simulink model "accelerate"  (R2022a)
settings: Solver=VariableStepAuto  StartTime=0.0  StopTime=2  FixedStep=0.0001  RelTol=1e-2  AbsTol=1e-2  EnableMultiTasking=on
InitFcn:
  | run('parameters.m')
  | run('initBusObjects.m')
  | run('loadTrajectory.m')
settings Model: Creator=chrismailer  LastModifiedBy=chrismailer
settings SolverCC: AutoScaleAbsTol=off  NumberNewtonIterations=3  ZeroCrossAlgorithm=Adaptive  AlgebraicLoopSolver=TrustRegion  AutoInsertRateTranBlk=on
settings DataIOCC: LimitDataPoints=on  MaxDataPoints=10000
settings OptimizationCC: LifeSpan=inf
settings DebuggingCC: UnconnectedInputMsg=warning  UnconnectedOutputMsg=warning  UnconnectedLineMsg=warning  AllowSymbolicDim=off  SFUnexpectedBacktrackingDiag=warning  SFNoUnconditionalDefaultTransitionDiag=warning  SFExecutionAtInitializationDiag=none  SFMachineParentedDataDiag=warning  ArithmeticOperatorsInVariantConditions=warning
settings SFSimCC: SimUseLocalCustomCode=off  CustomCodeUndefinedFunction=UseInterfaceOnly
settings RTWCC: RTWUseLocalCustomCode=off  DLArmComputeVersion=19.05
settings CodeAppCC: StateflowObjectComments=on
settings GRTTargetCC: TargetLangStandard=C89/C90 (ANSI)
settings ConfigComp: CovMetricSettings=dw  CovSaveCumulativeToWorkspaceVar=on  CovSaveSingleToWorkspaceVar=on  CovExternalEMLEnable=off  CovSFcnEnable=off
settings SimscapeCC: SimscapeLogType=all  SimscapeLogSimulationStatistics=on  SimscapeLogDataHistory=10000
settings ExplorerConfigSet: InternalSimMechanicsExplorerSettings="<ExplorerConfiguration><canonicalview>default</canonicalview><AnimationSetting><BasePlaybackSpeed>1.0</BasePlaybackSpeed><PlaybackSpeedFactor>0.125</PlaybackSpeedFactor></AnimationSetting><TilePanel><TileInfo><Tiles Columns=\"1\" Count=\"1\" Rows=\"1\"><Column Weight=\"1\"/><Row Weight=\"1\"/><Tile Height=\"1\" Width=\"1\" X=\"0\" Y=\"0\"/></Tiles></TileInfo><SceneInfo><SceneViewer><BGColor><R>1</R><G>1</G><B>1</B></BGColor><Camera><DoPerspective>on</DoPerspective><Position><X>3.29782276099316451</X><Y>0.285165922205473821</Y><Z>0.279114537761918247</Z></Position><Center><X>2.60042520557901913</X><Y>0.224861281402514157</Y><Z>0.27911453776191808</Z></Center><Up><X>0</X><Y>0</Y><Z>1</Z></Up><ViewLimDist>1</ViewLimDist><YLim>0.466307658154998583</YLim><XLim>0.737672809220199066</XLim></Camera></SceneViewer></SceneInfo></TilePanel><MechEditorPanel><Cameras><Camera><Id>Camera1</Id><Value><Name>Camera1</Name><NativeCamera><PositionTrackingFeature>Kemba_Simulation.Camera_Origin.R</PositionTrackingFeature><CenterTrackingFeature>Kemba_Simulation.Body.R</CenterTrackingFeature><UpVectorTrackingFeature>Kemba_Simulation.World_Frame.W</UpVectorTrackingFeature><CenterTrackingOrigin>on</CenterTrackingOrigin><UpVectorTrackingDirection>+Z</UpVectorTrackingDirection></NativeCamera></Value></Camera></Cameras><GfxPanelCameraMap><MapElement CameraMLId=\"Camera1\" GfxPanelIndex=\"0\"/></GfxPanelCameraMap><VideoCreator><PlaybackSpeedRatio>1.0</PlaybackSpeedRatio><FrameRate>30</FrameRate><VideoFormat>MPEG-4</VideoFormat><FrameSize>[1920 1080]</FrameSize></VideoCreator></MechEditorPanel></ExplorerConfiguration>"

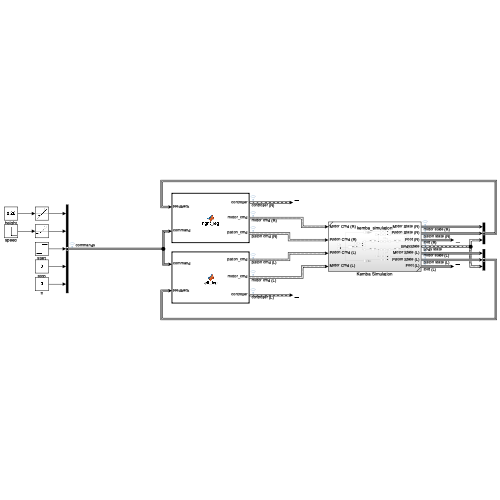
[thumbnail: Simulink's stored preview of the top-level diagram]
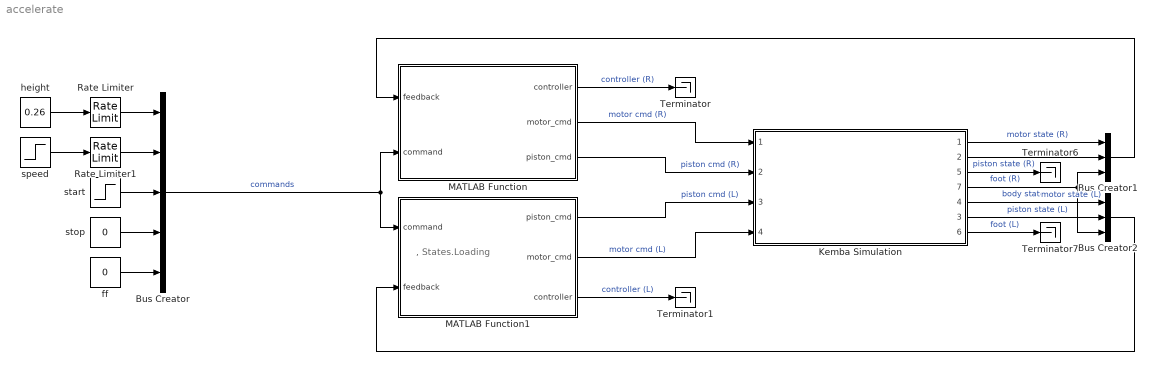
== system accelerate ==
  note: , States.Loading
  Bus Creator : BusCreator  Inputs=5  OutDataTypeStr=Bus: Command
      settings: InheritFromInputs=off
  Bus Creator1 : BusCreator  Inputs=3  OutDataTypeStr=Bus: State
      settings: InheritFromInputs=off
  Bus Creator2 : BusCreator  Inputs=3  OutDataTypeStr=Bus: State
      settings: InheritFromInputs=off
  Kemba Simulation : Subsystem  ReferencedSubsystem=kemba_simulation
      settings: PortSchema="{\"entries\":[{\"content\":{\"sides\":[{\"content\":{\"connectorIds\":[\"In1\",\"In2\",\"In3\",\"In4\"]},\"type\":\"ConnectorPlacement.EquallySpacedRectSide\",\"uuid\":\"35a785e7-99ad-4766-87e3-a239e5d8a8f8\"},{\"content\":{\"connectorIds\":[\"Out1\",\"Out2\",\"Out5\",\"Out7\",\"Out4\",\"Out3\",\"Out6\"],\"side\":\"RIGHT\"},\"type\":\"ConnectorPlacement.EquallySpacedRectSide\",\"uuid\":\"8c5f00f3-e1d5-4c02-a562-5da7bf8e4c30\"},{\"content\":{\"connectorIds\":[],\"side\":\"TOP\"},\"type\":\"ConnectorPlacement.EquallySpacedRectSide\",\"uuid\":\"cf7efd56-02a7-4dc2-b997-d6a0137d575f\"}]},\"type\":\"ConnectorPlacement.EquallySpacedConnector\",\"uuid\":\"7dd37b2d-e40a-4db8-86aa-8036efc7fb4f\"}],\"packageUris\":[\"http://schema.mathworks.com/mf0/Connector/R2020b\"],\"version\":\"1.0\"}"
  MATLAB Function : MATLAB Function  TreatAsAtomicUnit=on  SystemSampleTime=0.001
  MATLAB Function1 : MATLAB Function  TreatAsAtomicUnit=on  SystemSampleTime=0.001
  Rate Limiter : RateLimiter  RisingSlewLimit=0.05  FallingSlewLimit=-0.05  SampleTimeMode=inherited
  Rate Limiter1 : RateLimiter  RisingSlewLimit=0.4  FallingSlewLimit=-0.4  SampleTimeMode=inherited  InitialCondition=1.5
  Terminator{,1,6..7} (4 alike) : Terminator
  ff : Constant  Value=0
  height : Constant  Value=0.26
  speed : Step  Time=2  Before=1.5  After=0  SampleTime=0
  start : Step  Time=0.5  SampleTime=0
  stop : Constant  Value=0
  wires:
  MATLAB Function/2(motor_cmd) -> Kemba Simulation/1  "motor cmd (R)"
  Kemba Simulation/7 -> Bus Creator2/3, Bus Creator1/3  "body state"
  MATLAB Function/3(piston_cmd) -> Kemba Simulation/2  "piston cmd (R)"
  MATLAB Function1/2(motor_cmd) -> Kemba Simulation/4  "motor cmd (L)"
  MATLAB Function/1(controller) -> Terminator/1  "controller (R)"
  MATLAB Function1/3(controller) -> Terminator1/1  "controller (L)"
  height/1 -> Rate Limiter/1
  MATLAB Function1/1(piston_cmd) -> Kemba Simulation/3  "piston cmd (L)"
  Kemba Simulation/2 -> Bus Creator1/2  "piston state (R)"
  Kemba Simulation/1 -> Bus Creator1/1  "motor state (R)"
  Bus Creator1/1 -> MATLAB Function/1(feedback)
  Kemba Simulation/3 -> Bus Creator2/2  "piston state (L)"
  Kemba Simulation/4 -> Bus Creator2/1  "motor state (L)"
  Bus Creator2/1 -> MATLAB Function1/2(feedback)
  start/1 -> Bus Creator/3
  Kemba Simulation/5 -> Terminator6/1  "foot (R)"
  Kemba Simulation/6 -> Terminator7/1  "foot (L)"
  Rate Limiter/1 -> Bus Creator/1
  Bus Creator/1 -> MATLAB Function1/1(command), MATLAB Function/2(command)  "commands"
  ff/1 -> Bus Creator/5
  stop/1 -> Bus Creator/4
  speed/1 -> Rate Limiter1/1
  Rate Limiter1/1 -> Bus Creator/2

== matlab function accelerate/MATLAB Function ==
  data: controller output Bus: Controller; feedback input; motor_cmd output Bus: MotorCmd; piston_cmd output Bus: PistonCmd; command input Bus: Command
function [controller, motor_cmd, piston_cmd] = right_leg(feedback, command)

% initialisation
hip.y = 0; hip.dy = 0; hip.y_min = 0; hip.y_max = 0;
foot.y = 0; foot.height = 0; foot.contact = false; foot.radius = 20e-3;

motor = feedback.Motor;
piston = feedback.Piston;
body = feedback.Body;

% kinematics
[r,dr,phi,~] = virtural_leg_f(piston.v, body.dr, motor.w, piston.p, body.r, motor.q);
[~, ~ ,hip.y, hip.dy] = hip_pos_f(body.dr, body.dx, body.dy, body.r, body.x, body.y);
[~,foot.y] = foot_pos_f(piston.p, body.r, motor.q, body.x, body.y);

% constants
contact_threshold = 5e-3; % m relies on ground being flat
contact_acceleration_threshold = -100; % m/s^2
retract_duration = 17; % 17ms
hip.amplitude = 0.02;
hip.y_min = command.height - 0.5*hip.amplitude;
hip.y_max = command.height + 0.5*hip.amplitude;

persistent state
persistent retract_timer
persistent ground_offset
persistent Ts
if isempty(state)
    state = States.Rest;
end
if isempty(retract_timer)
    retract_timer = 0;
end
if isempty(ground_offset)
    ground_offset = 0;
end
if isempty(Ts)
    Ts = 0;
end
 
% contact detection
foot.height = foot.y + ground_offset;
if foot.height > contact_threshold
    foot.contact = false;
else
    foot.contact = true;
end
 
% state transitions
switch(state)
    case States.Rest
        if command.start
            ground_offset = -foot.y;
            state = States.Accelerate;
        end
    case States.Accelerate
        if hip.dy > 0
            if (hip.y + ground_offset) > ((hip.dy*hip.dy)/(-2*9.81) + hip.y_max)
                retract_timer = 0;
                ground_offset = -foot.y;
                state = States.Unloading;
            end
        end
    case States.Flight
        if ((hip.y + ground_offset) < ((2.5*hip.dy*hip.dy)/(2*50) + hip.y_min)) && (hip.dy < 0)
            state = States.Loading;
        elseif (hip.y_min < 0.17) && (command.stop)
            state = States.Rest;
        end
    case States.Loading
        if (piston.a < contact_acceleration_threshold) || (foot.contact)
            Ts = 0;
            state = States.Stance;
        end
    case States.Stance
        if hip.dy > 0
            if (hip.y + ground_offset) > ((hip.dy*hip.dy)/(-2*9.81) + hip.y_max)
                retract_timer = 0;
                ground_offset = -foot.y; % update ground offset
                state = States.Unloading;
            end
        end
    case States.Unloading
        if ~foot.contact
            state = States.Flight;
        end
end
 
 
% control piston
switch(state)
    case {States.Loading, States.Stance, States.Accelerate}
        piston_cmd.ue = 1;
        piston_cmd.ur = 0;
    case States.Unloading
        piston_cmd.ue = 0;
        if retract_timer < retract_duration
            piston_cmd.ur = 1;
        else
            piston_cmd.ur = 0;
        end
        retract_timer = retract_timer + 1;
    otherwise
        piston_cmd.ue = 0;
        piston_cmd.ur = 0;
end

% stance timer
switch(state)
    case {States.Stance, States.Unloading}
        Ts = Ts + 0.001;
end
 
% control motor
foot_offset = 0;
switch(state)
    case {States.Stance, States.Unloading, States.Loading}
        phi_d = -pi/2;
        dphi_d = (dr*cos(phi) + command.speed)/(r*sin(phi));
        Kp = 0;
        Kd = 4;
    case States.Accelerate
        phi_d = -pi/2;
        dphi_d = 0;
        Kp = 100;
        Kd = 4;
    case {States.Flight}
        foot_offset = (0.5*max(body.dx, command.speed)*(0.10))/r;
        foot_offset = max(min(foot_offset,1),-1);
        phi_d = -pi/2 + asin(foot_offset);
        dphi_d = 0;
        Kp = 100; % 80
        Kd = 4; % 2
    otherwise
        phi_d = -pi/2;
        dphi_d = 0;
        Kp = 50;
        Kd = 4;
end

[theta_m_des, dtheta_m_des] = phi_tracking_f(piston.v, dphi_d, body.dr, piston.p, phi_d, body.r);
% bound motor angle to not break pneumatics
theta_m_des = max(-pi, theta_m_des);

motor_cmd.q = theta_m_des;
motor_cmd.w = dtheta_m_des;
motor_cmd.Kp = Kp;
motor_cmd.Kd = Kd;
motor_cmd.tff = 0;

controller.state = state;
controller.Ts = Ts;
 
end

== matlab function accelerate/MATLAB Function1 ==
  data: command input Bus: Command; piston_cmd output Bus: PistonCmd; motor_cmd output Bus: MotorCmd; feedback input; controller output Bus: Controller
function [piston_cmd, motor_cmd, controller] = left_leg(command, feedback)

% initialisation
hip.y = 0; hip.dy = 0; hip.y_min = 0; hip.y_max = 0;
foot.y = 0; foot.height = 0; foot.contact = false; foot.radius = 20e-3;

% constants
contact_threshold = 5e-3; % m foot radius
contact_acceleration_threshold = -100; % m/s^2
retract_duration = 17; % 17ms
hip.amplitude = 0.02;
hip.y_min = command.height - 0.5*hip.amplitude;
hip.y_max = command.height + 0.5*hip.amplitude;

motor = feedback.Motor;
piston = feedback.Piston;
body = feedback.Body;

% kinematics
[r,dr,phi,~] = virtural_leg_b(piston.v, body.dr, motor.w, piston.p, body.r, motor.q);
[~, ~ ,hip.y, hip.dy] = hip_pos_b(body.dr, body.dx, body.dy, body.r, body.x, body.y);
[~,foot.y] = foot_pos_b(piston.p, body.r, motor.q, body.x, body.y);

persistent state
persistent retract_timer
persistent ground_offset
persistent Ts
if isempty(state)
    state = States.Rest;
end
if isempty(retract_timer)
    retract_timer = 0;
end
if isempty(ground_offset)
    ground_offset = 0;
end
if isempty(Ts)
    Ts = 0;
end

% contact detection
foot.height = foot.y + ground_offset;
if foot.height > contact_threshold
    foot.contact = false;
else
    foot.contact = true;
end

% state transitions
switch(state)
    case States.Rest
        if (body.r > 0.1) && (body.dr < 0) && (command.start) % wait until right leg has pushed off a bit
            state = States.Accelerate;
            ground_offset = -foot.y;
        end
    case States.Accelerate
        state = States.Stance;
    case States.Flight
        if ((hip.y + ground_offset) < ((2.5*hip.dy*hip.dy)/(2*50) + hip.y_min)) && (hip.dy < 0)
            state = States.Loading;
        elseif (hip.y_min < 0.17) && (command.stop)
            state = States.Rest;
        end
    case States.Loading
        if piston.a < contact_acceleration_threshold
            Ts = 0;
            state = States.Stance;
        end
    case States.Stance
        if hip.dy > 0
            if (hip.y + ground_offset) > ((hip.dy*hip.dy)/(-2*9.81) + hip.y_max)
                retract_timer = 0;
                ground_offset = -foot.y; % update ground offset
                state = States.Unloading;
            end
        end
    case States.Unloading
        if ~foot.contact
            state = States.Flight;
        end
end


% control piston
switch(state)
    case {States.Loading, States.Stance}
        piston_cmd.ue = 1;
        piston_cmd.ur = 0;
    case States.Unloading
        piston_cmd.ue = 0;
        if retract_timer < retract_duration
            piston_cmd.ur = 1;
        else
            piston_cmd.ur = 0;
        end
        retract_timer = retract_timer + 1;
    otherwise
        piston_cmd.ue = 0;
        piston_cmd.ur = 0;
end

% stance timer
switch(state)
    case {States.Stance, States.Unloading}
        Ts = Ts + 0.001;
end

% control motor
foot_offset = 0;
tff = 0;
switch(state)
    case {States.Stance, States.Unloading, States.Loading, States.Accelerate}
        phi_d = -pi/2;
        dphi_d = (dr*cos(phi) + command.speed)/(r*sin(phi));
        Kp = 0;
        Kd = 4;
    case {States.Flight}
        foot_offset = (0.5*max(body.dx, command.speed)*(0.10))/r;
        foot_offset = max(min(foot_offset,1),-1);
        phi_d = -pi/2 + asin(foot_offset);
        dphi_d = 0;
        Kp = 100; % 80
        Kd = 4; % 2
    case States.Rest
        foot_offset = (0.5*command.speed*(0.08))/r;
        foot_offset = max(min(foot_offset,1),-1);
        phi_d = -pi/2 + asin(foot_offset);
        dphi_d = 0;
        Kp = 50;
        Kd = 4;
    otherwise
        phi_d = -pi/2;
        dphi_d = 0;
        Kp = 50;
        Kd = 4;
end

[theta_m_des,dtheta_m_des] = phi_tracking_b(piston.v, dphi_d, body.dr, piston.p, phi_d, body.r);
% bound motor angle to not break pneumatics
theta_m_des =  min(theta_m_des, 0);

motor_cmd.q = theta_m_des;
motor_cmd.w = dtheta_m_des;
motor_cmd.Kp = Kp;
motor_cmd.Kd = Kd;
motor_cmd.tff = tff;

controller.state = state;
controller.Ts = Ts;
 
end
